simulink model "PenduloClase20240318"  (R2023b)
settings: Solver=VariableStepAuto  StartTime=0.0  StopTime=10.0  RelTol=1e-3
settings Model: Creator=agher  LastModifiedBy=AlejandroGhersin
settings DebuggingCC: UnconnectedInputMsg=warning  UnconnectedOutputMsg=warning  UnconnectedLineMsg=warning
settings ModelReferenceCC: EnableRefExpFcnMdlSchedulingChecks=on
settings RTWCC: DLArmComputeVersion=19.05

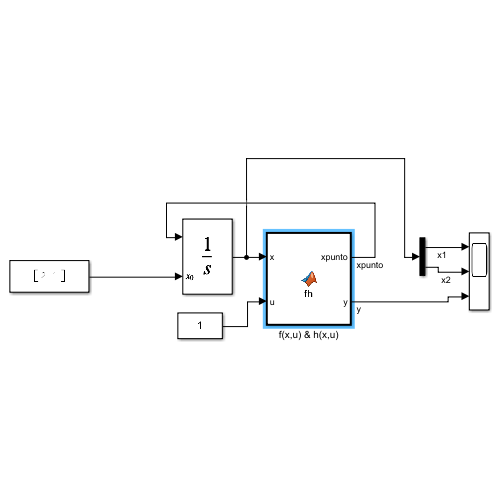
[thumbnail: Simulink's stored preview of the top-level diagram]
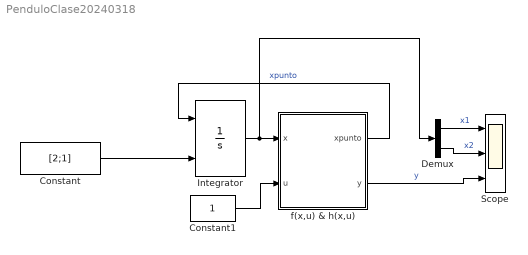
== system PenduloClase20240318 ==
  Constant : Constant  Value=[2;1]
  Constant1 : Constant
  Demux : Demux  Outputs=2
  Integrator : Integrator  InitialConditionSource=external
  Scope : Scope  NumInputPorts=3
  f(x,u) & h(x,u) : MATLAB Function  TreatAsAtomicUnit=on
  wires:
  f(x,u) & h(x,u)/1(xpunto) -> Integrator/1  "xpunto"
  Constant1/1 -> f(x,u) & h(x,u)/2(u)
  Constant/1 -> Integrator/2
  f(x,u) & h(x,u)/2(y) -> Scope/3  "y"
  Demux/1 -> Scope/1  "x1"
  Demux/2 -> Scope/2  "x2"
  Integrator/1 -> Demux/1, f(x,u) & h(x,u)/1(x)

== matlab function PenduloClase20240318/f(x,u) & h(x,u) ==
  data: x input; xpunto output; u input; y output
function [xpunto,y] = fh(x,u)

% f(x,u);
xpunto1=x(2);
xpunto2=- sin(x(1)) - 1*x(2) + u;

xpunto=[xpunto1;xpunto2];
% __________________
y = x(1); % h(x,u)
